simulink model "Model_1DoF_14b"  (R2014b)
settings: Solver=ode45  StartTime=0.0  StopTime=10.0  RelTol=1e-3
undefined symbols (not defined in the file or in its folder): in, param
settings Model: Creator=Zer0  LastModifiedBy=Arek

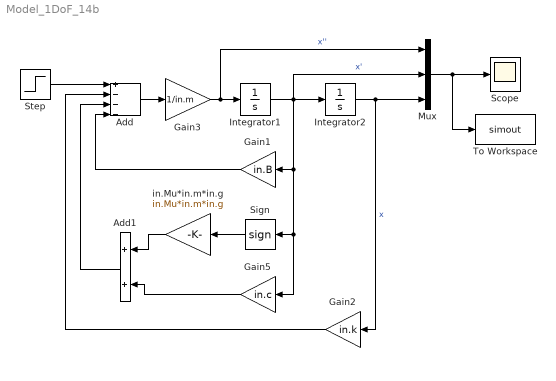
== system Model_1DoF_14b ==
  Add : Sum  Inputs=+---
  Add1 : Sum
  Gain1 : Gain  Gain=in.B
  Gain2 : Gain  Gain=in.k
  Gain3 : Gain  Gain=1/in.m
  Gain5 : Gain  Gain=in.c
  Integrator1 : Integrator  InitialCondition=param.ic(2)
  Integrator2 : Integrator  InitialCondition=param.ic(1)
  Mux : Mux  Inputs=3
  Scope : Scope
      settings: YMin=-0.8  YMax=0.8
  Sign : Signum  ZeroCross=off
  Step : Step  After=in.F  SampleTime=0
  To Workspace : ToWorkspace  VariableName=simout  SaveFormat=Timeseries  SampleTime=-1
  in.Mu*in.m*in.g : Gain  Gain=in.Mu*in.m*in.g
  wires:
  Integrator1/1 -> Mux/2, Gain1/1, Gain5/1, Sign/1, Integrator2/1  "x'"
  Gain1/1 -> Add/4
  Gain2/1 -> Add/2
  Integrator2/1 -> Gain2/1, Mux/3  "x"
  Mux/1 -> To Workspace/1, Scope/1
  Step/1 -> Add/1
  Add/1 -> Gain3/1
  Gain3/1 -> Mux/1, Integrator1/1  "x''"
  in.Mu*in.m*in.g/1 -> Add1/1
  Sign/1 -> in.Mu*in.m*in.g/1
  Add1/1 -> Add/3
  Gain5/1 -> Add1/2
